simulink model "sm_stewart_platform"  (R2019b)
settings: Solver=ode45  StartTime=0.0  StopTime=450  MaxStep=0.2  RelTol=1e-3  EnableMultiTasking=on
model workspace (MAT data in the model file):
  g_density = 5
values from neighbouring files (symbols this model uses):
  B = base_points.Data(:,:,1)    [run_this_for_sim.m]
  base_radius = 0.75*100    (= 75)    [run_this_for_sim.m]
  desired_max_angle = 10    [run_this_for_sim.m]
  desired_max_x = 0.05    [run_this_for_sim.m]
  desired_max_y = desired_max_x    (= 0.05)    [run_this_for_sim.m]
  desired_max_z = 0.05    [run_this_for_sim.m]
  initial_integral_force = 200    [run_this_for_sim.m]
  leg_max = leg_min+0.3    (= 1.322)    [run_this_for_sim.m]
  leg_min = 1.022    [run_this_for_sim.m]
  leg_thickness = 75/1000    (= 0.075)    [run_this_for_sim.m]
  lower_leg_length = upper_leg_length    (= 0.511)    [run_this_for_sim.m]
  max_velocity = 0.15    [run_this_for_sim.m]
  P = platform_points.Data(:,:,1)    [run_this_for_sim.m]
  platform_radius = 0.75*base_radius    (= 56.25)    [run_this_for_sim.m]
  platform_thickness = 0.1/8    (= 0.0125)    [run_this_for_sim.m]
  trajectory_smoothing = 1/1.5    (= 0.666666666667)    [run_this_for_sim.m]
  upper_leg_length = dead_length/2    (= 0.511)    [run_this_for_sim.m]
  work_height = 1.2*100    (= 120)    [run_this_for_sim.m]
undefined symbols (not defined in the file or in its folder): nom_length, X, Z
libraries: sp_lib x18, nesl_utility x11, sm_lib x9, simulink x2
(part 5 of 10)

== system sm_stewart_platform/Subsystem/Reference Trajectory Generator ==
  Clock : Clock
  Euler XYZ : Subsystem  mask(Euler XYZ){}
      mask help: Converts a set of Euler angles to the corresponding rotation matrix from rotated frame to fixed frame coordinates.
      mask Help:
      | An <em>Euler XYZ</em>  block converts a set of Euler angles to the corresponding
      |   rotation matrix from rotated frame to fixed frame coordinates.
      | 
      | Arbitrary 3-D rotations can be parameterized by a vector of three Euler angles:
      |   a, b, and c.  The resulting rotation is given by
      | 
      |     <b>R</b> = <b>R_x</b>(a) <b>R_y</b>(b) <b>R_z</b>(c).
      | 
      | where <b>R_x</b>, <b>R_y</b>, and <b>R_z</b> are rotations about the x, y, and z
      | axes, respectively.
      | 
      | The complete rotation <b>R</b> maps directions from a rotated frame F to a
      | fixed frame G.  Beginning with F and G in an aligned configuration, the full
      | rotation can be realized as a sequence of three rotations: first rotate F
      | about its x-axis, then rotate F about its y-axis, and finally rotate F about its
      | z-axis.  Alternatively, the rotation can be realized in a fixed-frame manner:
      | first rotate F about G's z-axis, then rotate F about G's y-axis, and finally
      | rotate F about G's z-axis.  Both interpretations are correct.
      | 
      | 
      | <h3>Ports</h3>
      | 
      | <ul>
      | 
      | <li> <b>angles</b> The Euler angles a, b, and c (in that order) as a 3-vector
      |   with units of radians.
      | 
      | <li> <b>R</b> The resulting rotation matrix.  This matrix is always a 3 x 3
      | orthogonal matrix with a +1 determinant.
      | 
      | </ul>
  Euler XYZ Derivative : Subsystem  mask(Euler XYZ Derivative){}
      mask help: Computes the first time derivative of a rotation matrix specified by a set of Euler angles.
      mask Help:
      | An <em>Euler XYZ Derivative</em>  block computes the first time derivative of a
      |  rotation matrix specified by a set of Euler angles.
      | 
      | Arbitrary 3-D rotations can be parameterized by a vector of three Euler angles:
      |   a, b, and c.  The resulting rotation is given by
      | 
      |     <b>R</b> = <b>R_x</b>(a) <b>R_y</b>(b) <b>R_z</b>(c).
      | 
      | where <b>R_x</b>, <b>R_y</b>, and <b>R_z</b> are rotations about the x, y, and z
      | axes, respectively.
      | 
      | If a, b, and c are, in turn, functions of time, with instantaneous derivatives
      | a', b', and c', then <b>R'</b>, the time derivative of <b>R</b> is given by
      | 
      |     <b>R'</b> = a' <b>i~ R_x</b>(a) <b>R_y</b>(b) <b>R_z</b>(c) + b' <b>R_x</b>(a) <b>j~ R_y</b>(b) <b>R_z</b>(c) + c' <b>R_x</b>(a) <b>R_y</b>(b) <b>k~ R_z</b>(c),
      | 
      | where <b>~</b> is the canonical operator converting a 3-vector <b>v</b> into a
      | corresponding 3 x 3 skew-symmetric matrix <b>v~</b> such that
      | 
      |     <b>v~ u</b> = <b>v</b> x <b>u</b> for all <b>u</b>.
      | 
      | With some vector algebra, the above expression of <b>R'</b> can be simplified to
      | 
      |     <b>R'</b> = [a' <b>i</b> + b' <b>R_x</b>(a) <b>j</b> ]<b>~</b> <b>R</b> + c' <b>[+R_2, -R_1, 0]</b>
      | 
      | where <b>R_i</b> is the ith column of <b>R</b>.
      | 
      | The block computes the value of <b>R'</b> according to the last equation above.
      | In addition to <b>R</b>, the computation requires the scalar Euler
      | angle <em>a</em>, and the time derivatives of all three Euler angles.
      | 
      | 
      | <h3>Ports</h3>
      | 
      | <ul>
      | 
      | <li> <b>R</b> The rotation matrix defined by the Euler angles <em>a, b,</em>
      | and <em>c</em> (see above).
      | 
      | <li> <b>a</b> The Euler angle corresponding to rotation about the x-axis.
      | 
      | <li> <b>a'</b> The time derivative of the Euler angle corresponding to rotation
      | about the x-axis.
      | 
      | <li> <b>b'</b> The time derivative of the Euler angle corresponding to rotation
      | about the y-axis.
      | 
      | <li> <b>c'</b> The time derivative of the Euler angle corresponding to rotation
      | about the z-axis.
      | 
      | </ul>
  Mux1 : Mux  Inputs=3
  Mux3 : Mux  Inputs=3
  Mux4 : Mux  Inputs=3
  Rx sinusoid : Subsystem  mask(Sinusoidal Trajectory){A=Aa * pi/180, w=wa, p=pa, k=ka * pi/180}
      mask prompts: A "Amplitude"; w "Frequency (deg / s)"; p "Phase (deg)"; k "Offset"
      mask help: Produces a time-varying sinusoid parameterized by amplitude, frequency, phase, and offset. Also produces the first time derivative of this function.
      mask Help:
      | A <em>Sinusoidal Trajectory</em> produces a time-varying sinusoid
      |  parameterized by amplitude, frequency, phase, and offset.  It also produces the
      |  first time derivative of this function.
      | 
      | <h3>Sinsoidal Functions</h3>
      | 
      | An arbitrary sinusoidal function of time and its first time derivative are given by
      | 
      |     f(t) = A sin (w t + p) + k
      |     f'(t) = w A cos (w t + p),
      | 
      | where <em>t</em> is time, and <em>A, w, p,</em> and <em>k</em> are scalar
      | constants.  Given time as an input signal, this block provides the f(t) and
      | f'(t) signals based on the parameters described above.
      | 
      | 
      | <h3>Parameters</h3>
      | 
      | The four parameters specify the scalar parameters described above:
      | 
      | <ul>
      | 
      | <li> <b>A</b> The <em>amplitude</em> of the sinusoid.
      | 
      | <li> <b>w</b> The <em>angular frequency</em> of the sinusoid.
      | 
      | <li> <b>p</b> The <em>phase</em> of the sinusoid.
      | 
      | <li> <b>k</b> The <em>offset</em> of the sinusoid.
      | 
      | </ul>
      | 
      | </ul>
      | 
      | <h3>Ports</h3>
      | 
      | <ul>
      | 
      | <li><b>t</b> The time function, provided as an input signal.
      | 
      | <li><b>f</b> The sinusoid f(t), as described above, as an output signal.
      | 
      | <li><b>f'</b> The sinusoid's first time derivative f'(t), as described above, as an output signal.
      | 
      | </ul>
  Ry sinusoid : Subsystem  mask(Sinusoidal Trajectory){A=Ab * pi/180, w=wb, p=pb, k=kb * pi/180}
      mask prompts: A "Amplitude"; w "Frequency (deg / s)"; p "Phase (deg)"; k "Offset"
      mask help: Produces a time-varying sinusoid parameterized by amplitude, frequency, phase, and offset. Also produces the first time derivative of this function.
      mask Help:
      | A <em>Sinusoidal Trajectory</em> produces a time-varying sinusoid
      |  parameterized by amplitude, frequency, phase, and offset.  It also produces the
      |  first time derivative of this function.
      | 
      | <h3>Sinsoidal Functions</h3>
      | 
      | An arbitrary sinusoidal function of time and its first time derivative are given by
      | 
      |     f(t) = A sin (w t + p) + k
      |     f'(t) = w A cos (w t + p),
      | 
      | where <em>t</em> is time, and <em>A, w, p,</em> and <em>k</em> are scalar
      | constants.  Given time as an input signal, this block provides the f(t) and
      | f'(t) signals based on the parameters described above.
      | 
      | 
      | <h3>Parameters</h3>
      | 
      | The four parameters specify the scalar parameters described above:
      | 
      | <ul>
      | 
      | <li> <b>A</b> The <em>amplitude</em> of the sinusoid.
      | 
      | <li> <b>w</b> The <em>angular frequency</em> of the sinusoid.
      | 
      | <li> <b>p</b> The <em>phase</em> of the sinusoid.
      | 
      | <li> <b>k</b> The <em>offset</em> of the sinusoid.
      | 
      | </ul>
      | 
      | </ul>
      | 
      | <h3>Ports</h3>
      | 
      | <ul>
      | 
      | <li><b>t</b> The time function, provided as an input signal.
      | 
      | <li><b>f</b> The sinusoid f(t), as described above, as an output signal.
      | 
      | <li><b>f'</b> The sinusoid's first time derivative f'(t), as described above, as an output signal.
      | 
      | </ul>
  Rz sinusoid : Subsystem  mask(Sinusoidal Trajectory){A=Ac * pi/180, w=wc, p=pc, k=kc * pi/180}
      mask prompts: A "Amplitude"; w "Frequency (deg / s)"; p "Phase (deg)"; k "Offset"
      mask help: Produces a time-varying sinusoid parameterized by amplitude, frequency, phase, and offset. Also produces the first time derivative of this function.
      mask Help:
      | A <em>Sinusoidal Trajectory</em> produces a time-varying sinusoid
      |  parameterized by amplitude, frequency, phase, and offset.  It also produces the
      |  first time derivative of this function.
      | 
      | <h3>Sinsoidal Functions</h3>
      | 
      | An arbitrary sinusoidal function of time and its first time derivative are given by
      | 
      |     f(t) = A sin (w t + p) + k
      |     f'(t) = w A cos (w t + p),
      | 
      | where <em>t</em> is time, and <em>A, w, p,</em> and <em>k</em> are scalar
      | constants.  Given time as an input signal, this block provides the f(t) and
      | f'(t) signals based on the parameters described above.
      | 
      | 
      | <h3>Parameters</h3>
      | 
      | The four parameters specify the scalar parameters described above:
      | 
      | <ul>
      | 
      | <li> <b>A</b> The <em>amplitude</em> of the sinusoid.
      | 
      | <li> <b>w</b> The <em>angular frequency</em> of the sinusoid.
      | 
      | <li> <b>p</b> The <em>phase</em> of the sinusoid.
      | 
      | <li> <b>k</b> The <em>offset</em> of the sinusoid.
      | 
      | </ul>
      | 
      | </ul>
      | 
      | <h3>Ports</h3>
      | 
      | <ul>
      | 
      | <li><b>t</b> The time function, provided as an input signal.
      | 
      | <li><b>f</b> The sinusoid f(t), as described above, as an output signal.
      | 
      | <li><b>f'</b> The sinusoid's first time derivative f'(t), as described above, as an output signal.
      | 
      | </ul>
  dx sinusoid : Subsystem  mask(Sinusoidal Trajectory){A=Ax, w=wx, p=px, k=kx}
      mask prompts: A "Amplitude"; w "Frequency (deg / s)"; p "Phase (deg)"; k "Offset"
      mask help: Produces a time-varying sinusoid parameterized by amplitude, frequency, phase, and offset. Also produces the first time derivative of this function.
      mask Help:
      | A <em>Sinusoidal Trajectory</em> produces a time-varying sinusoid
      |  parameterized by amplitude, frequency, phase, and offset.  It also produces the
      |  first time derivative of this function.
      | 
      | <h3>Sinsoidal Functions</h3>
      | 
      | An arbitrary sinusoidal function of time and its first time derivative are given by
      | 
      |     f(t) = A sin (w t + p) + k
      |     f'(t) = w A cos (w t + p),
      | 
      | where <em>t</em> is time, and <em>A, w, p,</em> and <em>k</em> are scalar
      | constants.  Given time as an input signal, this block provides the f(t) and
      | f'(t) signals based on the parameters described above.
      | 
      | 
      | <h3>Parameters</h3>
      | 
      | The four parameters specify the scalar parameters described above:
      | 
      | <ul>
      | 
      | <li> <b>A</b> The <em>amplitude</em> of the sinusoid.
      | 
      | <li> <b>w</b> The <em>angular frequency</em> of the sinusoid.
      | 
      | <li> <b>p</b> The <em>phase</em> of the sinusoid.
      | 
      | <li> <b>k</b> The <em>offset</em> of the sinusoid.
      | 
      | </ul>
      | 
      | </ul>
      | 
      | <h3>Ports</h3>
      | 
      | <ul>
      | 
      | <li><b>t</b> The time function, provided as an input signal.
      | 
      | <li><b>f</b> The sinusoid f(t), as described above, as an output signal.
      | 
      | <li><b>f'</b> The sinusoid's first time derivative f'(t), as described above, as an output signal.
      | 
      | </ul>
  dy sinusoid : Subsystem  mask(Sinusoidal Trajectory){A=Ay, w=wy, p=py, k=ky}
      mask prompts: A "Amplitude"; w "Frequency (deg / s)"; p "Phase (deg)"; k "Offset"
      mask help: Produces a time-varying sinusoid parameterized by amplitude, frequency, phase, and offset. Also produces the first time derivative of this function.
      mask Help:
      | A <em>Sinusoidal Trajectory</em> produces a time-varying sinusoid
      |  parameterized by amplitude, frequency, phase, and offset.  It also produces the
      |  first time derivative of this function.
      | 
      | <h3>Sinsoidal Functions</h3>
      | 
      | An arbitrary sinusoidal function of time and its first time derivative are given by
      | 
      |     f(t) = A sin (w t + p) + k
      |     f'(t) = w A cos (w t + p),
      | 
      | where <em>t</em> is time, and <em>A, w, p,</em> and <em>k</em> are scalar
      | constants.  Given time as an input signal, this block provides the f(t) and
      | f'(t) signals based on the parameters described above.
      | 
      | 
      | <h3>Parameters</h3>
      | 
      | The four parameters specify the scalar parameters described above:
      | 
      | <ul>
      | 
      | <li> <b>A</b> The <em>amplitude</em> of the sinusoid.
      | 
      | <li> <b>w</b> The <em>angular frequency</em> of the sinusoid.
      | 
      | <li> <b>p</b> The <em>phase</em> of the sinusoid.
      | 
      | <li> <b>k</b> The <em>offset</em> of the sinusoid.
      | 
      | </ul>
      | 
      | </ul>
      | 
      | <h3>Ports</h3>
      | 
      | <ul>
      | 
      | <li><b>t</b> The time function, provided as an input signal.
      | 
      | <li><b>f</b> The sinusoid f(t), as described above, as an output signal.
      | 
      | <li><b>f'</b> The sinusoid's first time derivative f'(t), as described above, as an output signal.
      | 
      | </ul>
  dz sinusoid : Subsystem  mask(Sinusoidal Trajectory){A=Az, w=wz, p=pz, k=kz}
      mask prompts: A "Amplitude"; w "Frequency (deg / s)"; p "Phase (deg)"; k "Offset"
      mask help: Produces a time-varying sinusoid parameterized by amplitude, frequency, phase, and offset. Also produces the first time derivative of this function.
      mask Help:
      | A <em>Sinusoidal Trajectory</em> produces a time-varying sinusoid
      |  parameterized by amplitude, frequency, phase, and offset.  It also produces the
      |  first time derivative of this function.
      | 
      | <h3>Sinsoidal Functions</h3>
      | 
      | An arbitrary sinusoidal function of time and its first time derivative are given by
      | 
      |     f(t) = A sin (w t + p) + k
      |     f'(t) = w A cos (w t + p),
      | 
      | where <em>t</em> is time, and <em>A, w, p,</em> and <em>k</em> are scalar
      | constants.  Given time as an input signal, this block provides the f(t) and
      | f'(t) signals based on the parameters described above.
      | 
      | 
      | <h3>Parameters</h3>
      | 
      | The four parameters specify the scalar parameters described above:
      | 
      | <ul>
      | 
      | <li> <b>A</b> The <em>amplitude</em> of the sinusoid.
      | 
      | <li> <b>w</b> The <em>angular frequency</em> of the sinusoid.
      | 
      | <li> <b>p</b> The <em>phase</em> of the sinusoid.
      | 
      | <li> <b>k</b> The <em>offset</em> of the sinusoid.
      | 
      | </ul>
      | 
      | </ul>
      | 
      | <h3>Ports</h3>
      | 
      | <ul>
      | 
      | <li><b>t</b> The time function, provided as an input signal.
      | 
      | <li><b>f</b> The sinusoid f(t), as described above, as an output signal.
      | 
      | <li><b>f'</b> The sinusoid's first time derivative f'(t), as described above, as an output signal.
      | 
      | </ul>
  d : Outport  VectorParamsAs1DForOutWhenUnconnected=off
  R : Outport  Port=2  VectorParamsAs1DForOutWhenUnconnected=off
  d' : Outport  Port=3  VectorParamsAs1DForOutWhenUnconnected=off
  R' : Outport  Port=4  VectorParamsAs1DForOutWhenUnconnected=off
  wires:
  dx sinusoid/1(f) -> Mux3/1
  dy sinusoid/1(f) -> Mux3/2
  dz sinusoid/1(f) -> Mux3/3
  dx sinusoid/2(f') -> Mux4/1
  dy sinusoid/2(f') -> Mux4/2
  dz sinusoid/2(f') -> Mux4/3
  Mux3/1 -> d/1  "d"
  Mux4/1 -> d'/1  "d'"
  Rx sinusoid/1(f) -> Mux1/1, Euler XYZ Derivative/2(a)
  Euler XYZ Derivative/1(R') -> R'/1  "R'"
  Clock/1 -> Ry sinusoid/1(t), Rz sinusoid/1(t), Rx sinusoid/1(t), dz sinusoid/1(t), dy sinusoid/1(t), dx sinusoid/1(t)
  Ry sinusoid/1(f) -> Mux1/2
  Rz sinusoid/1(f) -> Mux1/3
  Rx sinusoid/2(f') -> Euler XYZ Derivative/3(a')
  Ry sinusoid/2(f') -> Euler XYZ Derivative/4(b')
  Rz sinusoid/2(f') -> Euler XYZ Derivative/5(c')
  Mux1/1 -> Euler XYZ/1(angles)
  Euler XYZ/1(R) -> R/1, Euler XYZ Derivative/1(R)  "R"

== system sm_stewart_platform/Subsystem/Reference Trajectory Generator1 ==
  Clock : Clock
  Euler XYZ : Subsystem  mask(Euler XYZ){}
      mask help: Converts a set of Euler angles to the corresponding rotation matrix from rotated frame to fixed frame coordinates.
      mask Help:
      | An <em>Euler XYZ</em>  block converts a set of Euler angles to the corresponding
      |   rotation matrix from rotated frame to fixed frame coordinates.
      | 
      | Arbitrary 3-D rotations can be parameterized by a vector of three Euler angles:
      |   a, b, and c.  The resulting rotation is given by
      | 
      |     <b>R</b> = <b>R_x</b>(a) <b>R_y</b>(b) <b>R_z</b>(c).
      | 
      | where <b>R_x</b>, <b>R_y</b>, and <b>R_z</b> are rotations about the x, y, and z
      | axes, respectively.
      | 
      | The complete rotation <b>R</b> maps directions from a rotated frame F to a
      | fixed frame G.  Beginning with F and G in an aligned configuration, the full
      | rotation can be realized as a sequence of three rotations: first rotate F
      | about its x-axis, then rotate F about its y-axis, and finally rotate F about its
      | z-axis.  Alternatively, the rotation can be realized in a fixed-frame manner:
      | first rotate F about G's z-axis, then rotate F about G's y-axis, and finally
      | rotate F about G's z-axis.  Both interpretations are correct.
      | 
      | 
      | <h3>Ports</h3>
      | 
      | <ul>
      | 
      | <li> <b>angles</b> The Euler angles a, b, and c (in that order) as a 3-vector
      |   with units of radians.
      | 
      | <li> <b>R</b> The resulting rotation matrix.  This matrix is always a 3 x 3
      | orthogonal matrix with a +1 determinant.
      | 
      | </ul>
  Euler XYZ Derivative : Subsystem  mask(Euler XYZ Derivative){}
      mask help: Computes the first time derivative of a rotation matrix specified by a set of Euler angles.
      mask Help:
      | An <em>Euler XYZ Derivative</em>  block computes the first time derivative of a
      |  rotation matrix specified by a set of Euler angles.
      | 
      | Arbitrary 3-D rotations can be parameterized by a vector of three Euler angles:
      |   a, b, and c.  The resulting rotation is given by
      | 
      |     <b>R</b> = <b>R_x</b>(a) <b>R_y</b>(b) <b>R_z</b>(c).
      | 
      | where <b>R_x</b>, <b>R_y</b>, and <b>R_z</b> are rotations about the x, y, and z
      | axes, respectively.
      | 
      | If a, b, and c are, in turn, functions of time, with instantaneous derivatives
      | a', b', and c', then <b>R'</b>, the time derivative of <b>R</b> is given by
      | 
      |     <b>R'</b> = a' <b>i~ R_x</b>(a) <b>R_y</b>(b) <b>R_z</b>(c) + b' <b>R_x</b>(a) <b>j~ R_y</b>(b) <b>R_z</b>(c) + c' <b>R_x</b>(a) <b>R_y</b>(b) <b>k~ R_z</b>(c),
      | 
      | where <b>~</b> is the canonical operator converting a 3-vector <b>v</b> into a
      | corresponding 3 x 3 skew-symmetric matrix <b>v~</b> such that
      | 
      |     <b>v~ u</b> = <b>v</b> x <b>u</b> for all <b>u</b>.
      | 
      | With some vector algebra, the above expression of <b>R'</b> can be simplified to
      | 
      |     <b>R'</b> = [a' <b>i</b> + b' <b>R_x</b>(a) <b>j</b> ]<b>~</b> <b>R</b> + c' <b>[+R_2, -R_1, 0]</b>
      | 
      | where <b>R_i</b> is the ith column of <b>R</b>.
      | 
      | The block computes the value of <b>R'</b> according to the last equation above.
      | In addition to <b>R</b>, the computation requires the scalar Euler
      | angle <em>a</em>, and the time derivatives of all three Euler angles.
      | 
      | 
      | <h3>Ports</h3>
      | 
      | <ul>
      | 
      | <li> <b>R</b> The rotation matrix defined by the Euler angles <em>a, b,</em>
      | and <em>c</em> (see above).
      | 
      | <li> <b>a</b> The Euler angle corresponding to rotation about the x-axis.
      | 
      | <li> <b>a'</b> The time derivative of the Euler angle corresponding to rotation
      | about the x-axis.
      | 
      | <li> <b>b'</b> The time derivative of the Euler angle corresponding to rotation
      | about the y-axis.
      | 
      | <li> <b>c'</b> The time derivative of the Euler angle corresponding to rotation
      | about the z-axis.
      | 
      | </ul>
  Mux1 : Mux  Inputs=3
  Mux3 : Mux  Inputs=3
  Mux4 : Mux  Inputs=3
  Rx sinusoid : Subsystem  mask(Sinusoidal Trajectory){A=Aa * pi/180, w=wa, p=pa, k=ka * pi/180}
      mask prompts: A "Amplitude"; w "Frequency (deg / s)"; p "Phase (deg)"; k "Offset"
      mask help: Produces a time-varying sinusoid parameterized by amplitude, frequency, phase, and offset. Also produces the first time derivative of this function.
      mask Help:
      | A <em>Sinusoidal Trajectory</em> produces a time-varying sinusoid
      |  parameterized by amplitude, frequency, phase, and offset.  It also produces the
      |  first time derivative of this function.
      | 
      | <h3>Sinsoidal Functions</h3>
      | 
      | An arbitrary sinusoidal function of time and its first time derivative are given by
      | 
      |     f(t) = A sin (w t + p) + k
      |     f'(t) = w A cos (w t + p),
      | 
      | where <em>t</em> is time, and <em>A, w, p,</em> and <em>k</em> are scalar
      | constants.  Given time as an input signal, this block provides the f(t) and
      | f'(t) signals based on the parameters described above.
      | 
      | 
      | <h3>Parameters</h3>
      | 
      | The four parameters specify the scalar parameters described above:
      | 
      | <ul>
      | 
      | <li> <b>A</b> The <em>amplitude</em> of the sinusoid.
      | 
      | <li> <b>w</b> The <em>angular frequency</em> of the sinusoid.
      | 
      | <li> <b>p</b> The <em>phase</em> of the sinusoid.
      | 
      | <li> <b>k</b> The <em>offset</em> of the sinusoid.
      | 
      | </ul>
      | 
      | </ul>
      | 
      | <h3>Ports</h3>
      | 
      | <ul>
      | 
      | <li><b>t</b> The time function, provided as an input signal.
      | 
      | <li><b>f</b> The sinusoid f(t), as described above, as an output signal.
      | 
      | <li><b>f'</b> The sinusoid's first time derivative f'(t), as described above, as an output signal.
      | 
      | </ul>
  Ry sinusoid : Subsystem  mask(Sinusoidal Trajectory){A=Ab * pi/180, w=wb, p=pb, k=kb * pi/180}
      mask prompts: A "Amplitude"; w "Frequency (deg / s)"; p "Phase (deg)"; k "Offset"
      mask help: Produces a time-varying sinusoid parameterized by amplitude, frequency, phase, and offset. Also produces the first time derivative of this function.
      mask Help:
      | A <em>Sinusoidal Trajectory</em> produces a time-varying sinusoid
      |  parameterized by amplitude, frequency, phase, and offset.  It also produces the
      |  first time derivative of this function.
      | 
      | <h3>Sinsoidal Functions</h3>
      | 
      | An arbitrary sinusoidal function of time and its first time derivative are given by
      | 
      |     f(t) = A sin (w t + p) + k
      |     f'(t) = w A cos (w t + p),
      | 
      | where <em>t</em> is time, and <em>A, w, p,</em> and <em>k</em> are scalar
      | constants.  Given time as an input signal, this block provides the f(t) and
      | f'(t) signals based on the parameters described above.
      | 
      | 
      | <h3>Parameters</h3>
      | 
      | The four parameters specify the scalar parameters described above:
      | 
      | <ul>
      | 
      | <li> <b>A</b> The <em>amplitude</em> of the sinusoid.
      | 
      | <li> <b>w</b> The <em>angular frequency</em> of the sinusoid.
      | 
      | <li> <b>p</b> The <em>phase</em> of the sinusoid.
      | 
      | <li> <b>k</b> The <em>offset</em> of the sinusoid.
      | 
      | </ul>
      | 
      | </ul>
      | 
      | <h3>Ports</h3>
      | 
      | <ul>
      | 
      | <li><b>t</b> The time function, provided as an input signal.
      | 
      | <li><b>f</b> The sinusoid f(t), as described above, as an output signal.
      | 
      | <li><b>f'</b> The sinusoid's first time derivative f'(t), as described above, as an output signal.
      | 
      | </ul>
  Rz sinusoid : Subsystem  mask(Sinusoidal Trajectory){A=Ac * pi/180, w=wc, p=pc, k=kc * pi/180}
      mask prompts: A "Amplitude"; w "Frequency (deg / s)"; p "Phase (deg)"; k "Offset"
      mask help: Produces a time-varying sinusoid parameterized by amplitude, frequency, phase, and offset. Also produces the first time derivative of this function.
      mask Help:
      | A <em>Sinusoidal Trajectory</em> produces a time-varying sinusoid
      |  parameterized by amplitude, frequency, phase, and offset.  It also produces the
      |  first time derivative of this function.
      | 
      | <h3>Sinsoidal Functions</h3>
      | 
      | An arbitrary sinusoidal function of time and its first time derivative are given by
      | 
      |     f(t) = A sin (w t + p) + k
      |     f'(t) = w A cos (w t + p),
      | 
      | where <em>t</em> is time, and <em>A, w, p,</em> and <em>k</em> are scalar
      | constants.  Given time as an input signal, this block provides the f(t) and
      | f'(t) signals based on the parameters described above.
      | 
      | 
      | <h3>Parameters</h3>
      | 
      | The four parameters specify the scalar parameters described above:
      | 
      | <ul>
      | 
      | <li> <b>A</b> The <em>amplitude</em> of the sinusoid.
      | 
      | <li> <b>w</b> The <em>angular frequency</em> of the sinusoid.
      | 
      | <li> <b>p</b> The <em>phase</em> of the sinusoid.
      | 
      | <li> <b>k</b> The <em>offset</em> of the sinusoid.
      | 
      | </ul>
      | 
      | </ul>
      | 
      | <h3>Ports</h3>
      | 
      | <ul>
      | 
      | <li><b>t</b> The time function, provided as an input signal.
      | 
      | <li><b>f</b> The sinusoid f(t), as described above, as an output signal.
      | 
      | <li><b>f'</b> The sinusoid's first time derivative f'(t), as described above, as an output signal.
      | 
      | </ul>
  dx sinusoid : Subsystem  mask(Sinusoidal Trajectory){A=Ax, w=wx, p=px, k=kx}
      mask prompts: A "Amplitude"; w "Frequency (deg / s)"; p "Phase (deg)"; k "Offset"
      mask help: Produces a time-varying sinusoid parameterized by amplitude, frequency, phase, and offset. Also produces the first time derivative of this function.
      mask Help:
      | A <em>Sinusoidal Trajectory</em> produces a time-varying sinusoid
      |  parameterized by amplitude, frequency, phase, and offset.  It also produces the
      |  first time derivative of this function.
      | 
      | <h3>Sinsoidal Functions</h3>
      | 
      | An arbitrary sinusoidal function of time and its first time derivative are given by
      | 
      |     f(t) = A sin (w t + p) + k
      |     f'(t) = w A cos (w t + p),
      | 
      | where <em>t</em> is time, and <em>A, w, p,</em> and <em>k</em> are scalar
      | constants.  Given time as an input signal, this block provides the f(t) and
      | f'(t) signals based on the parameters described above.
      | 
      | 
      | <h3>Parameters</h3>
      | 
      | The four parameters specify the scalar parameters described above:
      | 
      | <ul>
      | 
      | <li> <b>A</b> The <em>amplitude</em> of the sinusoid.
      | 
      | <li> <b>w</b> The <em>angular frequency</em> of the sinusoid.
      | 
      | <li> <b>p</b> The <em>phase</em> of the sinusoid.
      | 
      | <li> <b>k</b> The <em>offset</em> of the sinusoid.
      | 
      | </ul>
      | 
      | </ul>
      | 
      | <h3>Ports</h3>
      | 
      | <ul>
      | 
      | <li><b>t</b> The time function, provided as an input signal.
      | 
      | <li><b>f</b> The sinusoid f(t), as described above, as an output signal.
      | 
      | <li><b>f'</b> The sinusoid's first time derivative f'(t), as described above, as an output signal.
      | 
      | </ul>
  dy sinusoid : Subsystem  mask(Sinusoidal Trajectory){A=Ay, w=wy, p=py, k=ky}
      mask prompts: A "Amplitude"; w "Frequency (deg / s)"; p "Phase (deg)"; k "Offset"
      mask help: Produces a time-varying sinusoid parameterized by amplitude, frequency, phase, and offset. Also produces the first time derivative of this function.
      mask Help:
      | A <em>Sinusoidal Trajectory</em> produces a time-varying sinusoid
      |  parameterized by amplitude, frequency, phase, and offset.  It also produces the
      |  first time derivative of this function.
      | 
      | <h3>Sinsoidal Functions</h3>
      | 
      | An arbitrary sinusoidal function of time and its first time derivative are given by
      | 
      |     f(t) = A sin (w t + p) + k
      |     f'(t) = w A cos (w t + p),
      | 
      | where <em>t</em> is time, and <em>A, w, p,</em> and <em>k</em> are scalar
      | constants.  Given time as an input signal, this block provides the f(t) and
      | f'(t) signals based on the parameters described above.
      | 
      | 
      | <h3>Parameters</h3>
      | 
      | The four parameters specify the scalar parameters described above:
      | 
      | <ul>
      | 
      | <li> <b>A</b> The <em>amplitude</em> of the sinusoid.
      | 
      | <li> <b>w</b> The <em>angular frequency</em> of the sinusoid.
      | 
      | <li> <b>p</b> The <em>phase</em> of the sinusoid.
      | 
      | <li> <b>k</b> The <em>offset</em> of the sinusoid.
      | 
      | </ul>
      | 
      | </ul>
      | 
      | <h3>Ports</h3>
      | 
      | <ul>
      | 
      | <li><b>t</b> The time function, provided as an input signal.
      | 
      | <li><b>f</b> The sinusoid f(t), as described above, as an output signal.
      | 
      | <li><b>f'</b> The sinusoid's first time derivative f'(t), as described above, as an output signal.
      | 
      | </ul>
  dz sinusoid : Subsystem  mask(Sinusoidal Trajectory){A=Az, w=wz, p=pz, k=kz}
      mask prompts: A "Amplitude"; w "Frequency (deg / s)"; p "Phase (deg)"; k "Offset"
      mask help: Produces a time-varying sinusoid parameterized by amplitude, frequency, phase, and offset. Also produces the first time derivative of this function.
      mask Help:
      | A <em>Sinusoidal Trajectory</em> produces a time-varying sinusoid
      |  parameterized by amplitude, frequency, phase, and offset.  It also produces the
      |  first time derivative of this function.
      | 
      | <h3>Sinsoidal Functions</h3>
      | 
      | An arbitrary sinusoidal function of time and its first time derivative are given by
      | 
      |     f(t) = A sin (w t + p) + k
      |     f'(t) = w A cos (w t + p),
      | 
      | where <em>t</em> is time, and <em>A, w, p,</em> and <em>k</em> are scalar
      | constants.  Given time as an input signal, this block provides the f(t) and
      | f'(t) signals based on the parameters described above.
      | 
      | 
      | <h3>Parameters</h3>
      | 
      | The four parameters specify the scalar parameters described above:
      | 
      | <ul>
      | 
      | <li> <b>A</b> The <em>amplitude</em> of the sinusoid.
      | 
      | <li> <b>w</b> The <em>angular frequency</em> of the sinusoid.
      | 
      | <li> <b>p</b> The <em>phase</em> of the sinusoid.
      | 
      | <li> <b>k</b> The <em>offset</em> of the sinusoid.
      | 
      | </ul>
      | 
      | </ul>
      | 
      | <h3>Ports</h3>
      | 
      | <ul>
      | 
      | <li><b>t</b> The time function, provided as an input signal.
      | 
      | <li><b>f</b> The sinusoid f(t), as described above, as an output signal.
      | 
      | <li><b>f'</b> The sinusoid's first time derivative f'(t), as described above, as an output signal.
      | 
      | </ul>
  d : Outport  VectorParamsAs1DForOutWhenUnconnected=off
  R : Outport  Port=2  VectorParamsAs1DForOutWhenUnconnected=off
  d' : Outport  Port=3  VectorParamsAs1DForOutWhenUnconnected=off
  R' : Outport  Port=4  VectorParamsAs1DForOutWhenUnconnected=off
  wires:
  dx sinusoid/1(f) -> Mux3/1
  dy sinusoid/1(f) -> Mux3/2
  dz sinusoid/1(f) -> Mux3/3
  dx sinusoid/2(f') -> Mux4/1
  dy sinusoid/2(f') -> Mux4/2
  dz sinusoid/2(f') -> Mux4/3
  Mux3/1 -> d/1  "d"
  Mux4/1 -> d'/1  "d'"
  Rx sinusoid/1(f) -> Mux1/1, Euler XYZ Derivative/2(a)
  Euler XYZ Derivative/1(R') -> R'/1  "R'"
  Clock/1 -> Ry sinusoid/1(t), Rz sinusoid/1(t), Rx sinusoid/1(t), dz sinusoid/1(t), dy sinusoid/1(t), dx sinusoid/1(t)
  Ry sinusoid/1(f) -> Mux1/2
  Rz sinusoid/1(f) -> Mux1/3
  Rx sinusoid/2(f') -> Euler XYZ Derivative/3(a')
  Ry sinusoid/2(f') -> Euler XYZ Derivative/4(b')
  Rz sinusoid/2(f') -> Euler XYZ Derivative/5(c')
  Mux1/1 -> Euler XYZ/1(angles)
  Euler XYZ/1(R) -> R/1, Euler XYZ Derivative/1(R)  "R"
